simulink model "streaming_icecast_visual"  (R2015a)
settings: Solver=FixedStepDiscrete  StartTime=0.0  StopTime=10000  FixedStep=0.1  RelTol=1e-3
settings Model: Creator=windor  LastModifiedBy=windor

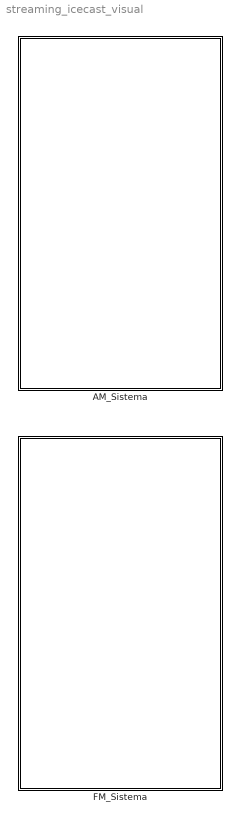
== system streaming_icecast_visual ==
  AM_Sistema : Subsystem
  FM_Sistema : Subsystem

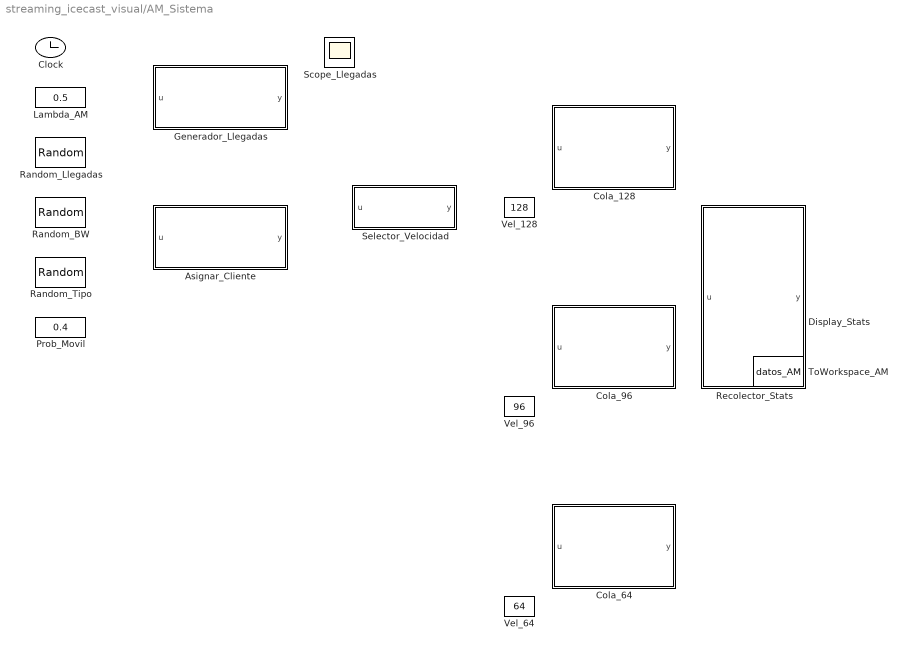
== system streaming_icecast_visual/AM_Sistema ==
  Asignar_Cliente : MATLAB Function  TreatAsAtomicUnit=on
  Clock : Clock
  Cola_128 : MATLAB Function  TreatAsAtomicUnit=on
  Cola_64 : MATLAB Function  TreatAsAtomicUnit=on
  Cola_96 : MATLAB Function  TreatAsAtomicUnit=on
  Display_Stats : Display
  Generador_Llegadas : MATLAB Function  TreatAsAtomicUnit=on
  Lambda_AM : Constant  Value=0.5
  Prob_Movil : Constant  Value=0.4
  Random_BW : UniformRandomNumber  Minimum=0  Seed=23456  SampleTime=0.1
  Random_Llegadas : UniformRandomNumber  Minimum=0  Seed=12345  SampleTime=0.1
  Random_Tipo : UniformRandomNumber  Minimum=0  Seed=34567  SampleTime=0.1
  Recolector_Stats : MATLAB Function  TreatAsAtomicUnit=on
  Scope_Llegadas : Scope
  Selector_Velocidad : MATLAB Function  TreatAsAtomicUnit=on
  ToWorkspace_AM : ToWorkspace  VariableName=datos_AM  SaveFormat=Structure  SampleTime=-1
  Vel_128 : Constant  Value=128
  Vel_64 : Constant  Value=64
  Vel_96 : Constant  Value=96

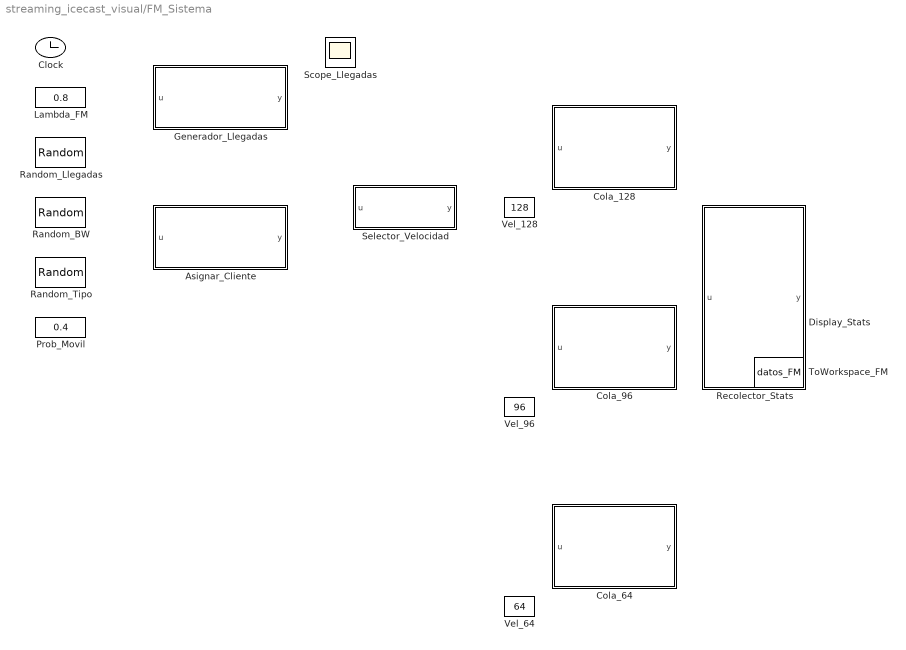
== system streaming_icecast_visual/FM_Sistema ==
  Asignar_Cliente : MATLAB Function  TreatAsAtomicUnit=on
  Clock : Clock
  Cola_128 : MATLAB Function  TreatAsAtomicUnit=on
  Cola_64 : MATLAB Function  TreatAsAtomicUnit=on
  Cola_96 : MATLAB Function  TreatAsAtomicUnit=on
  Display_Stats : Display
  Generador_Llegadas : MATLAB Function  TreatAsAtomicUnit=on
  Lambda_FM : Constant  Value=0.8
  Prob_Movil : Constant  Value=0.4
  Random_BW : UniformRandomNumber  Minimum=0  Seed=56789  SampleTime=0.1
  Random_Llegadas : UniformRandomNumber  Minimum=0  Seed=45678  SampleTime=0.1
  Random_Tipo : UniformRandomNumber  Minimum=0  Seed=67890  SampleTime=0.1
  Recolector_Stats : MATLAB Function  TreatAsAtomicUnit=on
  Scope_Llegadas : Scope
  Selector_Velocidad : MATLAB Function  TreatAsAtomicUnit=on
  ToWorkspace_FM : ToWorkspace  VariableName=datos_FM  SaveFormat=Structure  SampleTime=-1
  Vel_128 : Constant  Value=128
  Vel_64 : Constant  Value=64
  Vel_96 : Constant  Value=96

== matlab function streaming_icecast_visual/AM_Sistema/Asignar_Cliente ==
  data: u input; y output
function y = fcn(u)
%#codegen

y = u;

== matlab function streaming_icecast_visual/AM_Sistema/Generador_Llegadas ==
  data: u input; y output
function y = fcn(u)
%#codegen

y = u;

== matlab function streaming_icecast_visual/AM_Sistema/Selector_Velocidad ==
  data: u input; y output
function y = fcn(u)
%#codegen

y = u;

== matlab function streaming_icecast_visual/AM_Sistema/Cola_128 ==
  data: u input; y output
function y = fcn(u)
%#codegen

y = u;

== matlab function streaming_icecast_visual/AM_Sistema/Cola_96 ==
  data: u input; y output
function y = fcn(u)
%#codegen

y = u;

== matlab function streaming_icecast_visual/AM_Sistema/Cola_64 ==
  data: u input; y output
function y = fcn(u)
%#codegen

y = u;

== matlab function streaming_icecast_visual/AM_Sistema/Recolector_Stats ==
  data: u input; y output
function y = fcn(u)
%#codegen

y = u;

== matlab function streaming_icecast_visual/FM_Sistema/Generador_Llegadas ==
  data: u input; y output
function y = fcn(u)
%#codegen

y = u;

== matlab function streaming_icecast_visual/FM_Sistema/Asignar_Cliente ==
  data: u input; y output
function y = fcn(u)
%#codegen

y = u;

== matlab function streaming_icecast_visual/FM_Sistema/Selector_Velocidad ==
  data: u input; y output
function y = fcn(u)
%#codegen

y = u;

== matlab function streaming_icecast_visual/FM_Sistema/Cola_128 ==
  data: u input; y output
function y = fcn(u)
%#codegen

y = u;

== matlab function streaming_icecast_visual/FM_Sistema/Cola_96 ==
  data: u input; y output
function y = fcn(u)
%#codegen

y = u;

== matlab function streaming_icecast_visual/FM_Sistema/Cola_64 ==
  data: u input; y output
function y = fcn(u)
%#codegen

y = u;

== matlab function streaming_icecast_visual/FM_Sistema/Recolector_Stats ==
  data: u input; y output
function y = fcn(u)
%#codegen

y = u;
